simulink model "qxenv"  (Simulink 8.8)
settings: Solver=ode23tb  StartTime=0.0  StopTime=1  RelTol=1e-3  EnableMultiTasking=on
values from neighbouring files (symbols this model uses):
  Rr = 0.338    [Sphere.m]
undefined symbols (not defined in the file or in its folder): del_Rr, DiscIntNeverNeededParam
libraries: powerlib x4, powerlib_meascontrol x4, powerlib_extras x2, simulink x1
settings Model: SuppressorTable=22 serialization::archive 11 0 3 0 0 0 11 0  Creator=root  LastModifiedBy=root
settings DataIOCC: SignalLoggingSaveFormat=Dataset
settings DebuggingCC: UnderspecifiedInitializationDetection=Simplified  MergeDetectMultiDrivingBlocksExec=error  SolverPrmCheckMsg=warning  FcnCallInpInsideContextMsg=error  StateNameClashWarn=none
settings GRTTargetCC: CombineOutputUpdateFcns=on  GRTInterface=off
settings ConfigComp: CovSFcnEnable=off

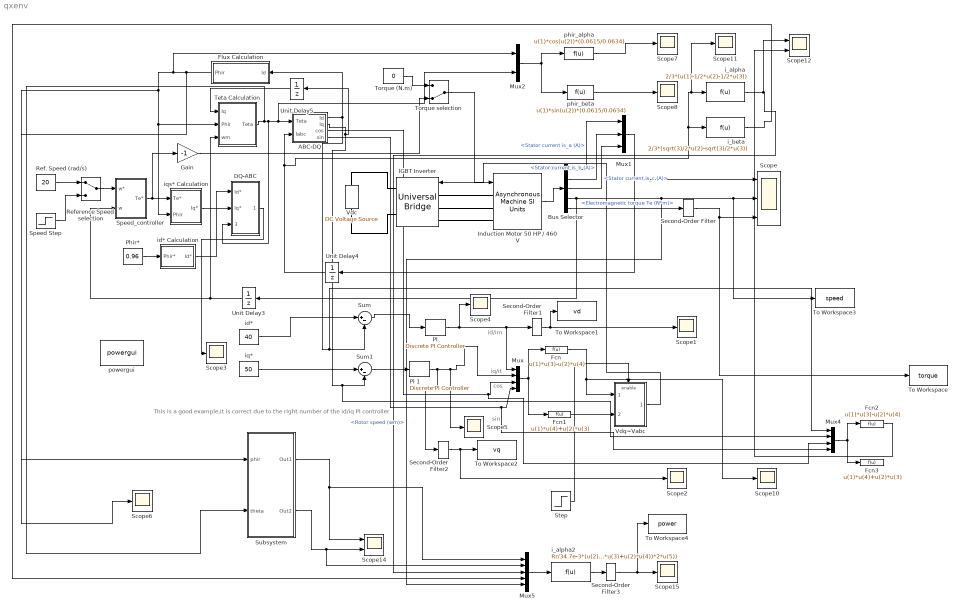
== system qxenv ==
  note: id/im
  note: iq/it
  note: cos
  note: sin
  note: This is a good example,it is correct due to the right number of the id/iq PI controller
  ABC-DQ : Subsystem
  Bus Selector : BusSelector  OutputSignals=Stator measurements.Stator current is_a (A),Stator measurements.Stator current is_b (A),Stator measurements.Stator current is_c (A),Mechanical.Rotor speed (wm),Mechanical.Electromagnetic torque Te (N*m)
  DQ-ABC : Subsystem
  Fcn : Fcn  Expr=u(1)*u(3)-u(2)*u(4)
  Fcn1 : Fcn  Expr=u(1)*u(4)+u(2)*u(3)
  Fcn2 : Fcn  Expr=u(1)*u(3)-u(2)*u(4)
  Fcn3 : Fcn  Expr=u(1)*u(4)+u(2)*u(3)
  Flux Calculation : Subsystem  mask(Flux Calcultation){}
      mask init:
      | NF=0.44572610323020e-6;
      | DF=[1 -0.99998715486734];
      mask Display: disp('Flux\nCalc.')
  Gain : Gain  Gain=-1
  IGBT Inverter : powerlib/Power Electronics/Universal Bridge  Arms=3  SnubberResistance=1000  SnubberCapacitance=inf  Device=IGBT / Diodes  Ron=1e-3  Lon=0  ForwardVoltages="[  0.8  0.8  ]"  ForwardVoltage=.8  GTOparameters=[ 1e-6 , 1e-6 ]  IGBTparameters=[ 1e-6 , 2e-6 ]  Measurements=None  Measurements_2=None  converterType=Rectifier
  Induction Motor 50 HP / 460 V : powerlib/Machines/Asynchronous Machine SI Units  RotorType=Squirrel-cage  PresetModel=No  MechanicalLoad=Torque Tm  ShowDetailedParameters=on  ReferenceFrame=Stationary  Units=SI  MeasurementBus=off  NominalParameters=[ 30000, 220, 50 ]  Stator=[ 0.087 0.8e-3 ]  Rotor=[ 0.328 0.8e-3 ]  Cage1=[ 0.022 0.226/377]  Cage2=[ 0.022 0.226/377]  Lm=34.7e-3  Mechanical="[3  0.1 2 ]"  PolePairs=2  InitialConditions="[ 1, 0 ,  0 , 0 , 0 , 0 , 0 , 0 ]"  SimulateSaturation=off  Saturation=[14.03593122, 27.81365428, 53.79336849, 72.68890987, 97.98006896, 148.6815601, 215.7428561, 302.9841135, 428.7778367 ; 230, 322, 414, 460, 506, 552, 598, 644, 690]  LoadFlowParameters=0  TsPowergui=0  TsBlock=-1  IterativeModel=Forward Euler  IterativeDiscreteModel=Trapezoidal non iterative  Pmec=0
  Mux : Mux
  Mux1 : Mux  Inputs=3
  Mux2 : Mux  Inputs=2
  Mux4 : Mux
  Mux5 : Mux  Inputs=5
  "PI " : powerlib_extras/Discrete  Control Blocks/Discrete PI Controller  Kp=20  Ki=20  Par_Limits=[600 -600]  Init=0  Ts=2e-6
  PI 1 : powerlib_extras/Discrete  Control Blocks/Discrete PI Controller  Kp=20  Ki=20  Par_Limits=[1800 -1800]  Init=0  Ts=2e-6
  Phir* : Constant  Value=0.96
  Ref. Speed (rad/s) : Constant  Value=20
  Reference Speed selection : ManualSwitch
  Scope : Scope  NumInputPorts=3
  Scope{1..8,10..11,15} (11 alike) : Scope
  Scope12 : Scope  NumInputPorts=2
  Scope14 : Scope  NumInputPorts=2
  Second-Order Filter{,1..3} (4 alike) : powerlib_meascontrol/Filters/Second-Order Filter  FilterType=Lowpass  Fo=5  Zeta=0.707  Ts=2e-6  Initialize=on  Vac_Init="[0,  0,  50]"  Vdc_Init=0  PlotResponse=off  FreqRange=[0, 500, 1]
  Speed Step : Step  Time=0.2  Before=120  After=160  SampleTime=0
  Speed_controller : Subsystem  mask(PI controller){Kp=3000, Ki=260, Tlim=30000, Ts=2e-6}
      mask prompts: Kp "Proportional gain (Kp)"; Ki "Integral gain (Ki)"; Tlim "Torque limit (N.m)"; Ts "Sampling time (s)"
      mask help: Proportional-Integral Speed Controller
      mask Display: plot(0,0,100,100,[35,35,65],[70,30,30],[35,65],[45,60])
  Step : Step  Time=0.2  SampleTime=0
  Subsystem : Subsystem
  Sum : Sum  Inputs=|+-  SaturateOnIntegerOverflow=on
  Sum1 : Sum  Inputs=|+-  SaturateOnIntegerOverflow=on
  Teta Calculation : Subsystem
  To Workspace : ToWorkspace  VariableName=torque  SampleTime=-1
      settings: Decimation=100
  To Workspace1 : ToWorkspace  VariableName=vd  SampleTime=-1
      settings: Decimation=100
  To Workspace2 : ToWorkspace  VariableName=vq  SampleTime=-1
      settings: Decimation=100
  To Workspace3 : ToWorkspace  VariableName=speed  SampleTime=-1
      settings: Decimation=100
  To Workspace4 : ToWorkspace  VariableName=power  SampleTime=-1
      settings: Decimation=100
  Torque selection : ManualSwitch  CurrentSetting=0
  Torque (N.m) : Constant  Value=0
  Unit Delay3 : UnitDelay  SampleTime=2e-6
  Unit Delay4 : UnitDelay  SampleTime=2e-6
  Unit Delay5 : UnitDelay  SampleTime=2e-6
  Vdc : powerlib/Electrical Sources/DC Voltage Source  Description=source block  Amplitude=1800  Measurements=None
      settings: AttributesFormatString=\n
  Vdq~Vabc : Subsystem
  i_alpha : Fcn  Expr=2/3*(u(1)-1/2*u(2)-1/2*u(3))
  i_alpha2 : Fcn  Expr=Rr/34.7e-3*(u(2)*u(3)-u(1)*u(4))-((u(1)*u(3)+u(2)*u(4))*2*u(5))
  i_beta : Fcn  Expr=2/3*(sqrt(3)/2*u(2)-sqrt(3)/2*u(3))
  id* : Constant  Value=40
  id* Calculation : Subsystem
  iq* : Constant  Value=50
  iqs* Calculation : Subsystem
  phir_alpha : Fcn  Expr=u(1)*cos(u(2))*(0.0615/0.0634)
  phir_beta : Fcn  Expr=u(1)*sin(u(2))*(0.0615/0.0634)
  powergui : powerlib/powergui  Priority=1  SimulationMode=Discrete  SolverType=Tustin  SampleTime=2e-6  frequency=60  SPID=off  DisableSnubberDevices=off  DisableRonSwitches=off  DisableVfSwitches=off  SwTol=0  DisplayEquations=off  Interpol=off  ExternalGateDelay=off  methode=off  Ts=0  FunctionMessages=off  echomessages=off  HookPort=off  EnableUseOfTLC=off  x0status=blocks  frequencyindice=50  Pbase=100e6  ErrMax=1e-4  Iterations=50  UnitsV=kV  UnitsW=MW  buscounter=0  RestoreLinks=warning  ResistiveCurrentMeasurement=off  Frange=[0:2:500]  Ylog=off  Xlog=on  ShowGrid=off  save=off  variable=ZData  structure=0  ZoomFFT=off  StartTime=0.0  cycles=1  DisplayStyle=1  fundamental=60  FreqAxis=off  MaxFrequency=1000  frequencyindicesteady=1  RmsSteady=1  display=off
  wires:
  Phir*/1 -> id* Calculation/1(Phir*)
  ABC-DQ/1(Id) -> Flux Calculation/1(Id), Mux4/1, Sum/2
  Unit Delay4/1 -> i_beta/1, Scope11/1, i_alpha/1, ABC-DQ/2(Iabc)
  Teta Calculation/1(Teta) -> Subsystem/2(theta), Mux2/2, ABC-DQ/1(Teta), DQ-ABC/3(Teta)
  iqs* Calculation/1(Iq*) -> DQ-ABC/2(Iq*)
  id* Calculation/1(Id*) -> DQ-ABC/1(Id*)
  Flux Calculation/1(Phir) -> Scope6/1, Mux2/1, Subsystem/1(phir), Teta Calculation/2(Phir), iqs* Calculation/2(Phir)
  Unit Delay3/1 -> Teta Calculation/3(wm), Speed_controller/2(w)
  ABC-DQ/2(Iq) -> Unit Delay5/1, Mux4/2, Sum1/2
  Unit Delay5/1 -> Teta Calculation/1(Iq)
  Vdq~Vabc/1(PWM) -> IGBT Inverter/1
  Speed_controller/1(Te*) -> Gain/1, iqs* Calculation/1(Te*)
  Torque (N.m)/1 -> Torque selection/1
  Torque selection/1 -> Induction Motor 50 HP / 460 V/1
  Ref. Speed (rad/s)/1 -> Reference Speed selection/1
  Speed Step/1 -> Reference Speed selection/2
  Reference Speed selection/1 -> Speed_controller/1(w*)
  Sum/1 -> "PI "/1
  Sum1/1 -> PI 1/1
  ABC-DQ/3(cos) -> Mux4/3, Mux/3
  ABC-DQ/4(sin) -> Mux4/4, Mux/4
  Mux/1 -> Fcn/1, Fcn1/1
  Fcn/1 -> Scope10/1, Vdq~Vabc/1(Valfa)
  Fcn1/1 -> Vdq~Vabc/2(Vbeta)
  iq*/1 -> Sum1/1
  Induction Motor 50 HP / 460 V/1 -> Bus Selector/1
  Bus Selector/1 -> Mux1/1  "<Stator current is_a (A)>"
  Bus Selector/2 -> Mux1/2  "<Stator current is_b (A)>"
  Bus Selector/3 -> Mux1/3  "<Stator current is_c (A)>"
  Mux1/1 -> Scope/1, Unit Delay4/1
  Bus Selector/4 -> Mux5/5, To Workspace3/1, Scope/2, Unit Delay3/1  "<Rotor speed (wm)>"
  Bus Selector/5 -> Second-Order Filter/1  "<Electromagnetic torque Te (N*m)>"
  id*/1 -> Sum/1
  DQ-ABC/1(Iabc*) -> Scope3/1
  Step/1 -> Vdq~Vabc/Enable
  Gain/1 -> Torque selection/2
  Second-Order Filter/1 -> To Workspace/1, Scope/3
  "PI "/1 -> Scope4/1, Second-Order Filter1/1, Mux/1
  PI 1/1 -> Scope5/1, Mux/2, Second-Order Filter2/1
  Second-Order Filter1/1 -> To Workspace1/1, Scope1/1
  Second-Order Filter2/1 -> Scope2/1, To Workspace2/1
  Mux2/1 -> phir_beta/1, phir_alpha/1
  phir_alpha/1 -> Scope7/1
  phir_beta/1 -> Scope8/1
  i_alpha/1 -> Scope12/1, Mux5/3
  i_beta/1 -> Mux5/4
  Mux4/1 -> Fcn3/1, Fcn2/1
  Fcn2/1 -> Scope12/2
  Subsystem/1(Out1) -> Mux5/1, Scope14/1
  Subsystem/2(Out2) -> Mux5/2, Scope14/2
  Mux5/1 -> i_alpha2/1
  i_alpha2/1 -> Second-Order Filter3/1
  Second-Order Filter3/1 -> To Workspace4/1, Scope15/1
  connections:
  IGBT Inverter/LConn3 -- Induction Motor 50 HP / 460 V/LConn3
  IGBT Inverter/RConn2 -- Vdc/LConn1
  Induction Motor 50 HP / 460 V/LConn1 -- IGBT Inverter/LConn1
  Induction Motor 50 HP / 460 V/LConn2 -- IGBT Inverter/LConn2
  Vdc/RConn1 -- IGBT Inverter/RConn1

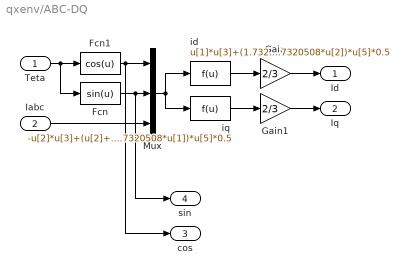
== system qxenv/ABC-DQ ==
  Teta : Inport
  Iabc : Inport  Port=2
  Fcn : Fcn  Expr=sin(u)
  Fcn1 : Fcn  Expr=cos(u)
  Gain : Gain  Gain=2/3  SaturateOnIntegerOverflow=on  OutDataTypeStr=Inherit: Same as input  ParamDataTypeStr=Inherit: Same as input
  Gain1 : Gain  Gain=2/3  SaturateOnIntegerOverflow=on  OutDataTypeStr=Inherit: Same as input  ParamDataTypeStr=Inherit: Same as input
  Mux : Mux  Inputs=[1 1 3]
  id : Fcn  Expr=u[1]*u[3]+(1.7320508*u[2]-u[1])*u[4]*0.5+(-u[1]-1.7320508*u[2])*u[5]*0.5
  iq : Fcn  Expr=-u[2]*u[3]+(u[2]+1.7320508*u[1])*u[4]*0.5+(u[2]-1.7320508*u[1])*u[5]*0.5
  Id : Outport  InitialOutput=0
  Iq : Outport  Port=2  InitialOutput=0
  cos : Outport  Port=3  InitialOutput=0
  sin : Outport  Port=4  InitialOutput=0
  wires:
  Fcn/1 -> Mux/2, sin/1
  Fcn1/1 -> Mux/1, cos/1
  Teta/1 -> Fcn1/1, Fcn/1
  Mux/1 -> iq/1, id/1
  Iabc/1 -> Mux/3
  iq/1 -> Gain1/1
  id/1 -> Gain/1
  Gain/1 -> Id/1
  Gain1/1 -> Iq/1

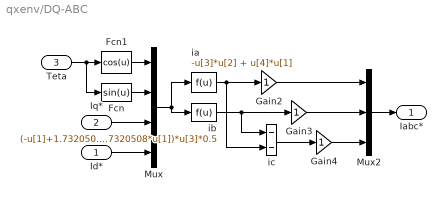
== system qxenv/DQ-ABC ==
  Id* : Inport
  Iq* : Inport  Port=2
  Teta : Inport  Port=3
  Fcn : Fcn  Expr=sin(u)
  Fcn1 : Fcn  Expr=cos(u)
  Gain2 : Gain  SaturateOnIntegerOverflow=on  OutDataTypeStr=Inherit: Same as input  ParamDataTypeStr=Inherit: Same as input
  Gain3 : Gain  SaturateOnIntegerOverflow=on  OutDataTypeStr=Inherit: Same as input  ParamDataTypeStr=Inherit: Same as input
  Gain4 : Gain  SaturateOnIntegerOverflow=on  OutDataTypeStr=Inherit: Same as input  ParamDataTypeStr=Inherit: Same as input
  Mux : Mux
  Mux2 : Mux  Inputs=3
  ia : Fcn  Expr=-u[3]*u[2] + u[4]*u[1]
  ib : Fcn  Expr=(-u[1]+1.7320508*u[2])*u[4]*0.5+(u[2]+1.7320508*u[1])*u[3]*0.5
  ic : Sum  Inputs=--  SaturateOnIntegerOverflow=on  InputSameDT=on  OutDataTypeStr=Inherit: Same as first input
  Iabc* : Outport  InitialOutput=0
  wires:
  Fcn/1 -> Mux/2
  Fcn1/1 -> Mux/1
  Mux2/1 -> Iabc*/1
  Mux/1 -> ib/1, ia/1
  Teta/1 -> Fcn1/1, Fcn/1
  Iq*/1 -> Mux/3
  Id*/1 -> Mux/4
  Gain3/1 -> Mux2/2
  ic/1 -> Gain4/1
  Gain4/1 -> Mux2/3
  Gain2/1 -> Mux2/1
  ia/1 -> Gain2/1, ic/2
  ib/1 -> Gain3/1, ic/1

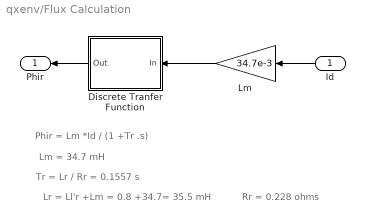
== system qxenv/Flux Calculation ==
  note: Phir = Lm *Id / (1 +Tr .s)
  note: Lm = 34.7 mH
  note: Lr = Ll'r +Lm = 0.8 +34.7= 35.5 mH
  note: Tr = Lr / Rr = 0.1557 s
  note: Rr = 0.228 ohms
  Id : Inport
  Discrete Tranfer Function : Subsystem  mask(First Order Low Pass Filter (Discrete)){T=35.5e-3/(Rr+del_Rr), Ts=2e-6}
      mask prompts: T "Time constant T (s) :"; Ts "Time step (s)"
      mask help: H(s)=1/(1+T.s)
      mask init:
      | X=[0 1 2 3 4];
      |  Y=[-2 -2 -3 -4 -4];
      |  str=sprintf('\nH=1/(1+T.s)\n T= %g s\n\n\n',T);
      | num=1;
      | den=[T 1];
      | 
      | % discrete transfer function
      | % descending powers of z
      | numd= Ts/T;
      | dend=[ 1  (Ts-T)/T];
      mask Display:
      | plot(X,Y);
      | disp(str);
  Lm : Gain  Gain=34.7e-3  SaturateOnIntegerOverflow=on  OutDataTypeStr=Inherit: Same as input  ParamDataTypeStr=Inherit: Same as input
  Phir : Outport
  wires:
  Discrete Tranfer Function/1(Out) -> Phir/1
  Id/1 -> Lm/1
  Lm/1 -> Discrete Tranfer Function/1(In)

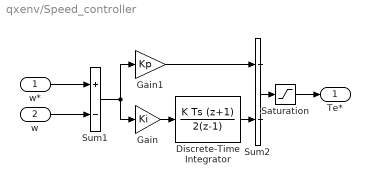
== system qxenv/Speed_controller ==
  w* : Inport
  w : Inport  Port=2
  Discrete-Time Integrator : DiscreteIntegrator  IntegratorMethod=Integration: Trapezoidal  SampleTime=Ts  LimitOutput=on  UpperSaturationLimit=Tlim  LowerSaturationLimit=-Tlim  ICPrevOutput=DiscIntNeverNeededParam  ICPrevScaledInput=DiscIntNeverNeededParam
  Gain : Gain  Gain=Ki  SaturateOnIntegerOverflow=on  OutDataTypeStr=Inherit: Same as input  ParamDataTypeStr=Inherit: Same as input
  Gain1 : Gain  Gain=Kp  SaturateOnIntegerOverflow=on  OutDataTypeStr=Inherit: Same as input  ParamDataTypeStr=Inherit: Same as input
  Saturation : Saturate  UpperLimit=Tlim  LowerLimit=-Tlim
  Sum1 : Sum  Inputs=+-  SaturateOnIntegerOverflow=on  InputSameDT=on  OutDataTypeStr=Inherit: Same as first input
  Sum2 : Sum  SaturateOnIntegerOverflow=on  InputSameDT=on  OutDataTypeStr=Inherit: Same as first input
  Te* : Outport  InitialOutput=0
  wires:
  Gain1/1 -> Sum2/1
  Gain/1 -> Discrete-Time Integrator/1
  Sum1/1 -> Gain/1, Gain1/1
  Discrete-Time Integrator/1 -> Sum2/2
  Sum2/1 -> Saturation/1
  Saturation/1 -> Te*/1
  w/1 -> Sum1/2
  w*/1 -> Sum1/1

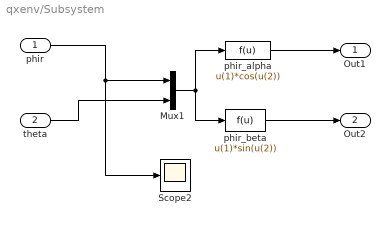
== system qxenv/Subsystem ==
  phir : Inport
  theta : Inport  Port=2
  Mux1 : Mux  Inputs=2
  Scope2 : Scope
  phir_alpha : Fcn  Expr=u(1)*cos(u(2))
  phir_beta : Fcn  Expr=u(1)*sin(u(2))
  Out1 : Outport
  Out2 : Outport  Port=2
  wires:
  phir/1 -> Mux1/1, Scope2/1
  Mux1/1 -> phir_alpha/1, phir_beta/1
  theta/1 -> Mux1/2
  phir_alpha/1 -> Out1/1
  phir_beta/1 -> Out2/1

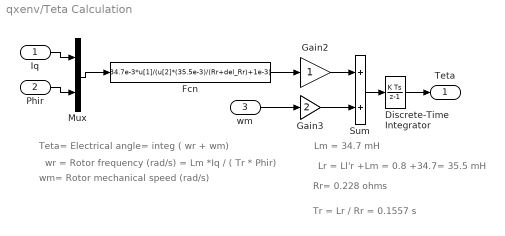
== system qxenv/Teta Calculation ==
  note: Teta= Electrical angle= integ ( wr + wm)
  note: wr = Rotor frequency (rad/s) = Lm *Iq / ( Tr * Phir)
  note: Lm = 34.7 mH
  note: Rr= 0.228 ohms
  note: Lr = Ll'r +Lm = 0.8 +34.7= 35.5 mH
  note: wm= Rotor mechanical speed (rad/s)
  note: Tr = Lr / Rr = 0.1557 s
  Iq : Inport
  Phir : Inport  Port=2
  wm : Inport  Port=3
  Discrete-Time Integrator : DiscreteIntegrator  SampleTime=2e-6  ICPrevOutput=DiscIntNeverNeededParam  ICPrevScaledInput=DiscIntNeverNeededParam
  Fcn : Fcn  Expr=34.7e-3*u[1]/(u[2]*(35.5e-3)/(Rr+del_Rr)+1e-3)
  Gain2 : Gain  SaturateOnIntegerOverflow=on  OutDataTypeStr=Inherit: Same as input  ParamDataTypeStr=Inherit: Same as input
  Gain3 : Gain  Gain=2  SaturateOnIntegerOverflow=on  OutDataTypeStr=Inherit: Same as input  ParamDataTypeStr=Inherit: Same as input
  Mux : Mux  Inputs=2
  Sum : Sum  SaturateOnIntegerOverflow=on  InputSameDT=on  OutDataTypeStr=Inherit: Same as first input
  Teta : Outport  InitialOutput=0
  wires:
  Discrete-Time Integrator/1 -> Teta/1
  Sum/1 -> Discrete-Time Integrator/1
  Gain3/1 -> Sum/2
  Gain2/1 -> Sum/1
  wm/1 -> Gain3/1
  Fcn/1 -> Gain2/1
  Phir/1 -> Mux/2
  Iq/1 -> Mux/1
  Mux/1 -> Fcn/1

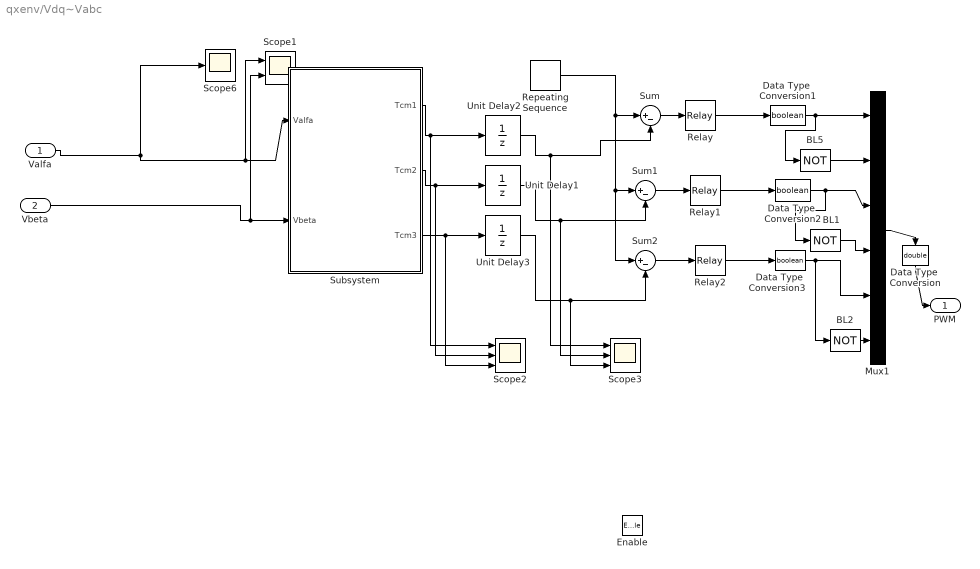
== system qxenv/Vdq~Vabc ==
  Valfa : Inport
  Vbeta : Inport  Port=2
  Enable : EnablePort
  BL1 : Logic  Operator=NOT  Inputs=1
  BL2 : Logic  Operator=NOT  Inputs=1
  BL5 : Logic  Operator=NOT  Inputs=1
  Data Type  Conversion : DataTypeConversion  OutDataTypeStr=double  SaturateOnIntegerOverflow=on  RndMeth=Zero
  Data Type  Conversion1 : DataTypeConversion  OutDataTypeStr=boolean  SaturateOnIntegerOverflow=on  RndMeth=Zero
  Data Type  Conversion2 : DataTypeConversion  OutDataTypeStr=boolean  SaturateOnIntegerOverflow=on  RndMeth=Zero
  Data Type  Conversion3 : DataTypeConversion  OutDataTypeStr=boolean  SaturateOnIntegerOverflow=on  RndMeth=Zero
  Mux1 : Mux  Inputs=6
  Relay : Relay  OnSwitchValue=1e-8  OffSwitchValue=-1e-8
  Relay1 : Relay  OnSwitchValue=1e-8  OffSwitchValue=-1e-8
  Relay2 : Relay  OnSwitchValue=1e-8  OffSwitchValue=-1e-8
  Repeating Sequence : simulink/Sources/Repeating Sequence  rep_seq_t=[0 0.00005 0.0001]  rep_seq_y=[0 0.00005 0]
  Scope1 : Scope  NumInputPorts=2
  Scope2 : Scope  NumInputPorts=3
  Scope3 : Scope  NumInputPorts=3
  Scope6 : Scope
  Subsystem : Subsystem
  Sum : Sum  Inputs=|+-  SaturateOnIntegerOverflow=on
  Sum1 : Sum  Inputs=|+-  SaturateOnIntegerOverflow=on
  Sum2 : Sum  Inputs=|+-  SaturateOnIntegerOverflow=on
  Unit Delay1 : UnitDelay  SampleTime=0.0001
  Unit Delay2 : UnitDelay  SampleTime=0.0001
  Unit Delay3 : UnitDelay  SampleTime=0.0001
  PWM : Outport
  wires:
  Repeating Sequence/1 -> Sum/1, Sum1/1, Sum2/1
  Sum/1 -> Relay/1
  Sum1/1 -> Relay1/1
  Sum2/1 -> Relay2/1
  Relay/1 -> Data Type  Conversion1/1
  Relay1/1 -> Data Type  Conversion2/1
  Relay2/1 -> Data Type  Conversion3/1
  Data Type  Conversion3/1 -> Mux1/5, BL2/1
  Data Type  Conversion2/1 -> BL1/1, Mux1/3
  Data Type  Conversion1/1 -> Mux1/1, BL5/1
  BL5/1 -> Mux1/2
  BL1/1 -> Mux1/4
  BL2/1 -> Mux1/6
  Subsystem/3(Tcm3) -> Unit Delay3/1, Scope2/3
  Subsystem/2(Tcm2) -> Unit Delay1/1, Scope2/2
  Mux1/1 -> Data Type  Conversion/1
  Data Type  Conversion/1 -> PWM/1
  Subsystem/1(Tcm1) -> Unit Delay2/1, Scope2/1
  Unit Delay2/1 -> Sum/2, Scope3/1
  Unit Delay1/1 -> Sum1/2, Scope3/2
  Unit Delay3/1 -> Sum2/2, Scope3/3
  Valfa/1 -> Scope6/1, Subsystem/1(Valfa), Scope1/1
  Vbeta/1 -> Subsystem/2(Vbeta), Scope1/2

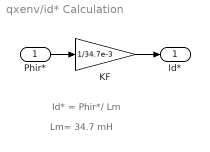
== system qxenv/id* Calculation ==
  note: Id* = Phir*/ Lm
  note: Lm= 34.7 mH
  Phir* : Inport
  KF : Gain  Gain=1/34.7e-3  SaturateOnIntegerOverflow=on  OutDataTypeStr=Inherit: Same as input  ParamDataTypeStr=Inherit: Same as input
  Id* : Outport
  wires:
  KF/1 -> Id*/1
  Phir*/1 -> KF/1

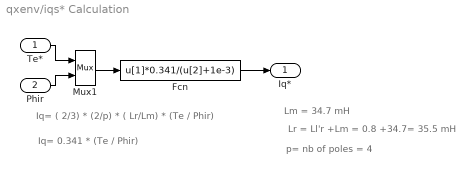
== system qxenv/iqs* Calculation ==
  note: Iq= ( 2/3) * (2/p) * ( Lr/Lm) * (Te / Phir)
  note: Lm = 34.7 mH
  note: Lr = Ll'r +Lm = 0.8 +34.7= 35.5 mH
  note: p= nb of poles = 4
  note: Iq= 0.341 * (Te / Phir)
  Te* : Inport
  Phir : Inport  Port=2
  Fcn : Fcn  Expr=u[1]*0.341/(u[2]+1e-3)
  Mux1 : Mux  Inputs=2
  Iq* : Outport  InitialOutput=0
  wires:
  Phir/1 -> Mux1/2
  Fcn/1 -> Iq*/1
  Te*/1 -> Mux1/1
  Mux1/1 -> Fcn/1

== system qxenv/Flux Calculation/Discrete Tranfer Function ==
  In : Inport
  Discrete Transfer Fcn : DiscreteTransferFcn  Numerator=numd  Denominator=dend  SampleTime=Ts
  Out : Outport  InitialOutput=0
  wires:
  Discrete Transfer Fcn/1 -> Out/1
  In/1 -> Discrete Transfer Fcn/1

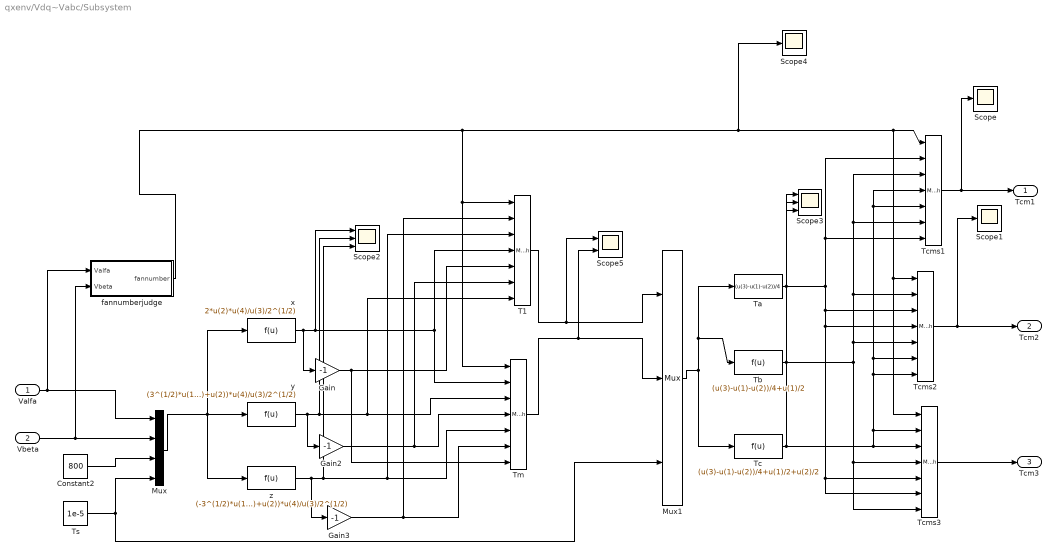
== system qxenv/Vdq~Vabc/Subsystem ==
  Valfa : Inport
  Vbeta : Inport  Port=2
  Constant2 : Constant  Value=800
  Gain : Gain  Gain=-1  SaturateOnIntegerOverflow=on  OutDataTypeStr=Inherit: Same as input  ParamDataTypeStr=Inherit: Same as input
  Gain2 : Gain  Gain=-1  SaturateOnIntegerOverflow=on  OutDataTypeStr=Inherit: Same as input  ParamDataTypeStr=Inherit: Same as input
  Gain3 : Gain  Gain=-1  SaturateOnIntegerOverflow=on  OutDataTypeStr=Inherit: Same as input  ParamDataTypeStr=Inherit: Same as input
  Mux : Mux
  Mux1 : Mux  Inputs=3
  Scope : Scope
  Scope1 : Scope
  Scope2 : Scope  NumInputPorts=3
  Scope3 : Scope  NumInputPorts=3
  Scope4 : Scope
  Scope5 : Scope  NumInputPorts=2
  T1 : MultiPortSwitch  Inputs=6  SaturateOnIntegerOverflow=on
  Ta : Fcn  Expr=(u(3)-u(1)-u(2))/4
  Tb : Fcn  Expr=(u(3)-u(1)-u(2))/4+u(1)/2
  Tc : Fcn  Expr=(u(3)-u(1)-u(2))/4+u(1)/2+u(2)/2
  Tcms1 : MultiPortSwitch  Inputs=6  SaturateOnIntegerOverflow=on
  Tcms2 : MultiPortSwitch  Inputs=6  SaturateOnIntegerOverflow=on
  Tcms3 : MultiPortSwitch  Inputs=6  SaturateOnIntegerOverflow=on
  Tm : MultiPortSwitch  Inputs=6  SaturateOnIntegerOverflow=on
  Ts : Constant  Value=1e-5
  fannumberjudge : Subsystem
  x : Fcn  Expr=2*u(2)*u(4)/u(3)/2^(1/2)
  y : Fcn  Expr=(3^(1/2)*u(1)+u(2))*u(4)/u(3)/2^(1/2)
  z : Fcn  Expr=(-3^(1/2)*u(1)+u(2))*u(4)/u(3)/2^(1/2)
  Tcm1 : Outport
  Tcm2 : Outport  Port=2
  Tcm3 : Outport  Port=3
  wires:
  Valfa/1 -> fannumberjudge/1(Valfa), Mux/1
  Vbeta/1 -> Mux/2, fannumberjudge/2(Vbeta)
  Tcms1/1 -> Tcm1/1, Scope/1
  fannumberjudge/1(fannumber) -> T1/1, Tm/1, Tcms1/1, Tcms2/1, Tcms3/1, Scope4/1
  Tcms2/1 -> Tcm2/1, Scope1/1
  Tcms3/1 -> Tcm3/1
  Mux/1 -> x/1, y/1, z/1
  Ts/1 -> Mux/4, Mux1/3
  Constant2/1 -> Mux/3
  z/1 -> Gain3/1, T1/3, Tm/5, Scope2/3
  Gain3/1 -> T1/2, Tm/6
  x/1 -> Gain/1, Tm/2, T1/4, Scope2/1
  y/1 -> Gain2/1, Tm/3, T1/7, Scope2/2
  Gain2/1 -> Tm/4, T1/6
  Gain/1 -> T1/5, Tm/7
  Mux1/1 -> Ta/1, Tb/1, Tc/1
  Ta/1 -> Tcms2/3, Tcms2/4, Tcms3/5, Tcms3/6, Tcms1/2, Tcms1/7, Scope3/1
  Tb/1 -> Tcms2/2, Tcms1/3, Tcms1/6, Tcms2/5, Tcms3/4, Tcms3/7, Scope3/2
  Tc/1 -> Tcms3/3, Tcms3/2, Tcms1/4, Tcms1/5, Tcms2/6, Tcms2/7, Scope3/3
  T1/1 -> Mux1/1, Scope5/1
  Tm/1 -> Mux1/2, Scope5/2

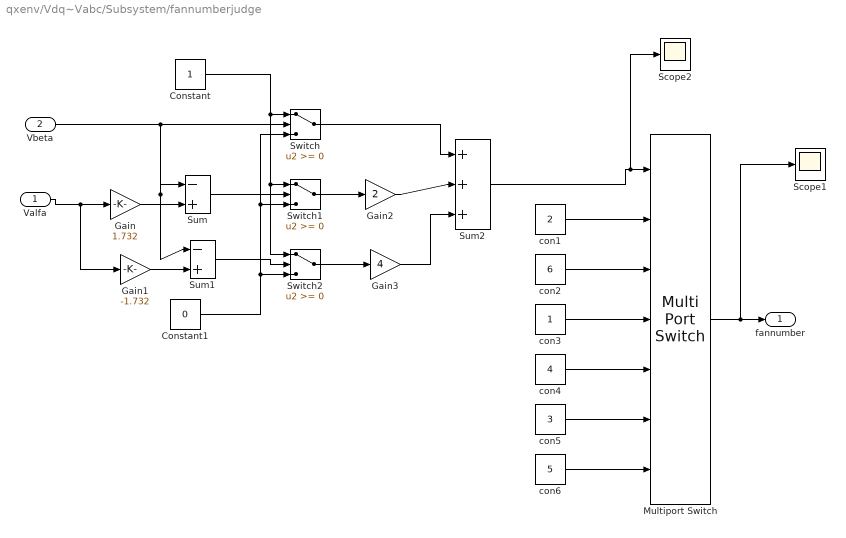
== system qxenv/Vdq~Vabc/Subsystem/fannumberjudge ==
  Valfa : Inport
  Vbeta : Inport  Port=2
  Constant : Constant
  Constant1 : Constant  Value=0
  Gain : Gain  Gain=1.732  SaturateOnIntegerOverflow=on  OutDataTypeStr=Inherit: Same as input  ParamDataTypeStr=Inherit: Same as input
  Gain1 : Gain  Gain=-1.732  SaturateOnIntegerOverflow=on  OutDataTypeStr=Inherit: Same as input  ParamDataTypeStr=Inherit: Same as input
  Gain2 : Gain  Gain=2  SaturateOnIntegerOverflow=on  OutDataTypeStr=Inherit: Same as input  ParamDataTypeStr=Inherit: Same as input
  Gain3 : Gain  Gain=4  SaturateOnIntegerOverflow=on  OutDataTypeStr=Inherit: Same as input  ParamDataTypeStr=Inherit: Same as input
  Multiport Switch : MultiPortSwitch  Inputs=6  SaturateOnIntegerOverflow=on
  Scope1 : Scope
  Scope2 : Scope
  Sum : Sum  Inputs=|-+  SaturateOnIntegerOverflow=on
  Sum1 : Sum  Inputs=|-+  SaturateOnIntegerOverflow=on
  Sum2 : Sum  Inputs=|+++  SaturateOnIntegerOverflow=on
  Switch : Switch  SaturateOnIntegerOverflow=on
  Switch1 : Switch  SaturateOnIntegerOverflow=on
  Switch2 : Switch  SaturateOnIntegerOverflow=on
  con1 : Constant  Value=2
  con2 : Constant  Value=6
  con3 : Constant
  con4 : Constant  Value=4
  con5 : Constant  Value=3
  con6 : Constant  Value=5
  fannumber : Outport
  wires:
  Multiport Switch/1 -> fannumber/1, Scope1/1
  con1/1 -> Multiport Switch/2
  con2/1 -> Multiport Switch/3
  con3/1 -> Multiport Switch/4
  con4/1 -> Multiport Switch/5
  con5/1 -> Multiport Switch/6
  con6/1 -> Multiport Switch/7
  Sum2/1 -> Multiport Switch/1, Scope2/1
  Gain3/1 -> Sum2/3
  Gain2/1 -> Sum2/2
  Switch/1 -> Sum2/1
  Switch2/1 -> Gain3/1
  Switch1/1 -> Gain2/1
  Gain1/1 -> Sum1/2
  Gain/1 -> Sum/2
  Valfa/1 -> Gain/1, Gain1/1
  Sum1/1 -> Switch2/2
  Sum/1 -> Switch1/2
  Constant1/1 -> Switch2/3, Switch1/3, Switch/3
  Constant/1 -> Switch1/1, Switch2/1, Switch/1
  Vbeta/1 -> Switch/2, Sum/1, Sum1/1
